simulink model "MSFartoystyring"  (R2019a)
settings: Solver=ode45  StartTime=tstart  StopTime=tstop  RelTol=1e-3  EnableMultiTasking=on
values from neighbouring files (symbols this model uses):
  c = 0    [run.m]
  p0 = zeros(2,1)    [run.m]
  psi0 = 0    [run.m]
  r0 = 0    [run.m]
  tsamp = 10    [run.m]
  v0 = [6.63 0]'    [run.m]
undefined symbols (not defined in the file or in its folder): dc_mode, delta_c, K_d_psi, K_d_u, K_i_psi, K_i_u, K_p_psi, K_p_u, k_reg, msfartoystyring, nc_mode, nc_step_final, nc_step_start, nc_step_time, psi_d_amp, psi_d_bias, psi_d_freq, r_reg, u_d_step_final, u_d_step_start, u_d_step_time
settings Model: ExtModeAutoUpdateStatusClock=off  Creator=christh  LastModifiedBy=paalthorseth
settings DataIOCC: LimitDataPoints=on  SaveFormat=Array  SignalLoggingSaveFormat=ModelDataLogs  ReturnWorkspaceOutputs=off
settings OptimizationCC: ExpressionDepthLimit=2147483647  InitFltsAndDblsToZero=on  LifeSpan=inf
settings DebuggingCC: UnderspecifiedInitializationDetection=Classic  MergeDetectMultiDrivingBlocksExec=none  SolverPrmCheckMsg=warning  FcnCallInpInsideContextMsg=warning  StateNameClashWarn=warning  SFUnexpectedBacktrackingDiag=warning  SFNoUnconditionalDefaultTransitionDiag=warning  ArithmeticOperatorsInVariantConditions=warning
settings HardwareCC: ProdBitPerPointer=32  ProdBitPerSizeT=32  ProdBitPerPtrDiffT=32  ProdLargestAtomicFloat=None  ProdIntDivRoundTo=Undefined  ProdEndianess=Unspecified  ProdWordSize=32  ProdHWDeviceType=32-bit Generic
settings ModelReferenceCC: PropagateSignalLabelsOutOfModel=off
settings SFSimCC: SimUseLocalCustomCode=off
settings RTWCC: RTWUseLocalCustomCode=off
settings CodeAppCC: StateflowObjectComments=on
settings GRTTargetCC: TargetLangStandard=C89/C90 (ANSI)  GeneratePreprocessorConditionals=Disable all  CombineOutputUpdateFcns=off  GRTInterface=on
settings ConfigComp: CovMetricSettings=dw  CovHtmlReporting=on  CovSaveCumulativeToWorkspaceVar=on  CovSaveSingleToWorkspaceVar=on  CovExternalEMLEnable=off

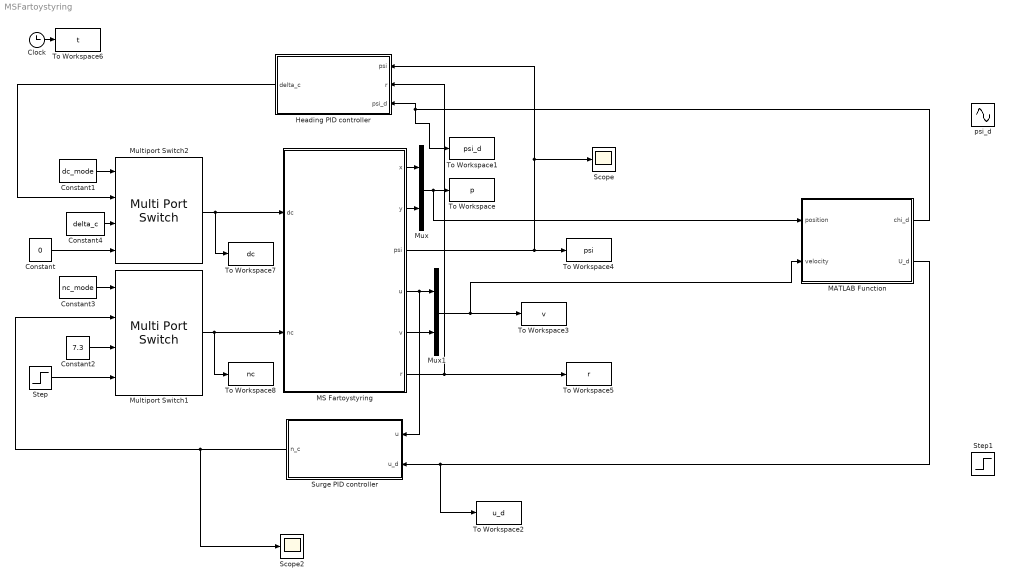
== system MSFartoystyring ==
  Clock : Clock
  Constant : Constant  Value=0
  Constant1 : Constant  Value=dc_mode
  Constant2 : Constant  Value=7.3
  Constant3 : Constant  Value=nc_mode
  Constant4 : Constant  Value=delta_c
  Heading PID controller : Subsystem
  MATLAB Function : MATLAB Function  TreatAsAtomicUnit=on  SystemSampleTime=0.1
  MS Fartoystyring : Subsystem  mask(MS Fartoystyring for Assignment 3 G&C){x0=p0(1), y0=p0(2), u0=v0(1), v0=v0(2), psi0=psi0, r0=r0, c=c}
      mask prompts: x0 "x(t0) (m)"; y0 "y(t0) (m)"; u0 "u(t0) (m/s)"; v0 "v(t0) (m/s)"; psi0 "psi(t0) (rad)"; r0 "r(t0) (rad/s)"; c "current (0 or 1)"
      mask help:
      | Block corresponding to Figure 1 in the assignment text. Gives the response of the ship.
      |
      | The design speed of MS Fartoystyring is u=8.23 m/s.
      |
      | Input:
      | dc: commanded rudder (rad), dmax=25*pi/180
      | nc: commanded shaft speed (rad/s), nmax=85*2*pi/60
      |
      | Output:
      | x: north pos (m)
      | y: east pos (m)
      | u: surge (m/s)
      | v: sway (m/s)
      | psi: heading (rad)
      | r: yaw (rad/s)
      mask Help: Comments, bugs and help requests can be directed to the TA. Email on course website.
  Multiport Switch1 : MultiPortSwitch  DataPortOrder=Specify indices  DataPortIndices={NC_MODE.CONTROLLER, NC_MODE.CONSTANT, NC_MODE.STEP}  DiagnosticForDefault=None
  Multiport Switch2 : MultiPortSwitch  DataPortOrder=Specify indices  DataPortIndices={DC_MODE.CONTROLLER, DC_MODE.CONSTANT, DC_MODE.ZERO}
  Mux : Mux  Inputs=2
  Mux1 : Mux  Inputs=2
  Scope : Scope
  Scope2 : Scope
  Step : Step  Time=nc_step_time  Before=nc_step_start  After=nc_step_final  SampleTime=0
  Step1 : Step  Time=u_d_step_time  Before=u_d_step_start  After=u_d_step_final  SampleTime=0
  Surge PID controller : Subsystem
  To Workspace : ToWorkspace  VariableName=p  SampleTime=tsamp
  To Workspace1 : ToWorkspace  VariableName=psi_d  SampleTime=tsamp
  To Workspace2 : ToWorkspace  VariableName=u_d  SampleTime=tsamp
  To Workspace3 : ToWorkspace  VariableName=v  SampleTime=tsamp
  To Workspace4 : ToWorkspace  VariableName=psi  SampleTime=tsamp
  To Workspace5 : ToWorkspace  VariableName=r  SampleTime=tsamp
  To Workspace6 : ToWorkspace  VariableName=t  SampleTime=tsamp
  To Workspace7 : ToWorkspace  VariableName=dc  SampleTime=tsamp
  To Workspace8 : ToWorkspace  VariableName=nc  SampleTime=tsamp
  psi_d : Sin  Amplitude=psi_d_amp  Bias=psi_d_bias  Frequency=psi_d_freq  SampleTime=0
  wires:
  Clock/1 -> To Workspace6/1
  MS Fartoystyring/1(x) -> Mux/1
  MS Fartoystyring/2(y) -> Mux/2
  MS Fartoystyring/5(v) -> Mux1/2
  MS Fartoystyring/3(psi) -> To Workspace4/1, Heading PID controller/1(psi), Scope/1
  MS Fartoystyring/6(r) -> To Workspace5/1, Heading PID controller/2(r)
  MATLAB Function/1(chi_d) -> To Workspace1/1, Heading PID controller/3(psi_d)
  Step/1 -> Multiport Switch1/4
  Constant2/1 -> Multiport Switch1/3
  Constant1/1 -> Multiport Switch2/1
  Constant3/1 -> Multiport Switch1/1
  Constant/1 -> Multiport Switch2/4
  Constant4/1 -> Multiport Switch2/3
  Heading PID controller/1(delta_c) -> Multiport Switch2/2
  Surge PID controller/1(n_c) -> Scope2/1, Multiport Switch1/2
  Multiport Switch2/1 -> To Workspace7/1, MS Fartoystyring/1(dc)
  Multiport Switch1/1 -> MS Fartoystyring/2(nc), To Workspace8/1
  MATLAB Function/2(U_d) -> Surge PID controller/2(u_d), To Workspace2/1
  MS Fartoystyring/4(u) -> Surge PID controller/1(u), Mux1/1
  Mux/1 -> MATLAB Function/1(position), To Workspace/1
  Mux1/1 -> MATLAB Function/2(velocity), To Workspace3/1

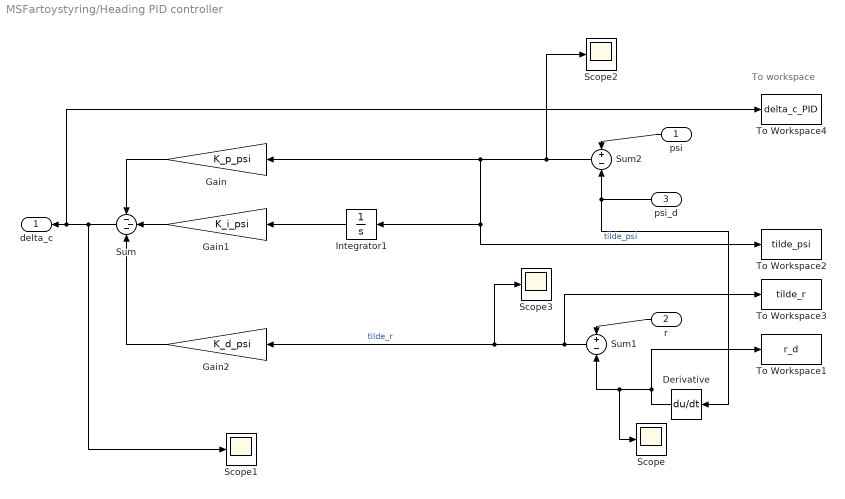
== system MSFartoystyring/Heading PID controller ==
  note: To workspace
  psi : Inport
  r : Inport  Port=2
  psi_d : Inport  Port=3
  Derivative : Derivative
  Gain : Gain  Gain=K_p_psi
  Gain1 : Gain  Gain=K_i_psi
  Gain2 : Gain  Gain=K_d_psi
  Integrator1 : Integrator
  Scope{,1..3} (4 alike) : Scope
  Sum : Sum  Inputs=---
  Sum1 : Sum  Inputs=+|-
  Sum2 : Sum  Inputs=+|-
  To Workspace1 : ToWorkspace  VariableName=r_d  SampleTime=tsamp
  To Workspace2 : ToWorkspace  VariableName=tilde_psi  SampleTime=tsamp
  To Workspace3 : ToWorkspace  VariableName=tilde_r  SampleTime=tsamp
  To Workspace4 : ToWorkspace  VariableName=delta_c_PID  SampleTime=tsamp
  delta_c : Outport
  wires:
  Sum/1 -> Scope1/1, delta_c/1, To Workspace4/1
  Gain/1 -> Sum/1
  Sum2/1 -> Scope2/1, Integrator1/1, To Workspace2/1, Gain/1  "tilde_psi"
  Derivative/1 -> Scope/1, Sum1/2, To Workspace1/1
  Integrator1/1 -> Gain1/1
  r/1 -> Sum1/1
  Sum1/1 -> Scope3/1, Gain2/1, To Workspace3/1  "tilde_r"
  psi/1 -> Sum2/1
  psi_d/1 -> Derivative/1, Sum2/2
  Gain2/1 -> Sum/3
  Gain1/1 -> Sum/2

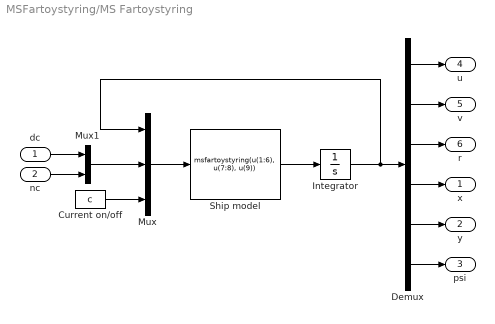
== system MSFartoystyring/MS Fartoystyring ==
  dc : Inport
  nc : Inport  Port=2
  Current on/off : Constant  Value=c
  Demux : Demux  Outputs=6
  Integrator : Integrator  InitialCondition=[u0 v0 r0 x0 y0 psi0]'
  Mux : Mux  Inputs=3
  Mux1 : Mux  Inputs=2
  Ship model : MATLABFcn  MATLABFcn=msfartoystyring(u(1:6), u(7:8), u(9))  OutputDimensions=6
  x : Outport
  y : Outport  Port=2
  psi : Outport  Port=3
  u : Outport  Port=4
  v : Outport  Port=5
  r : Outport  Port=6
  wires:
  Integrator/1 -> Mux/1, Demux/1
  Mux1/1 -> Mux/2
  dc/1 -> Mux1/1
  nc/1 -> Mux1/2
  Demux/1 -> u/1
  Demux/2 -> v/1
  Demux/3 -> r/1
  Demux/4 -> x/1
  Demux/5 -> y/1
  Demux/6 -> psi/1
  Current on/off/1 -> Mux/3
  Ship model/1 -> Integrator/1
  Mux/1 -> Ship model/1

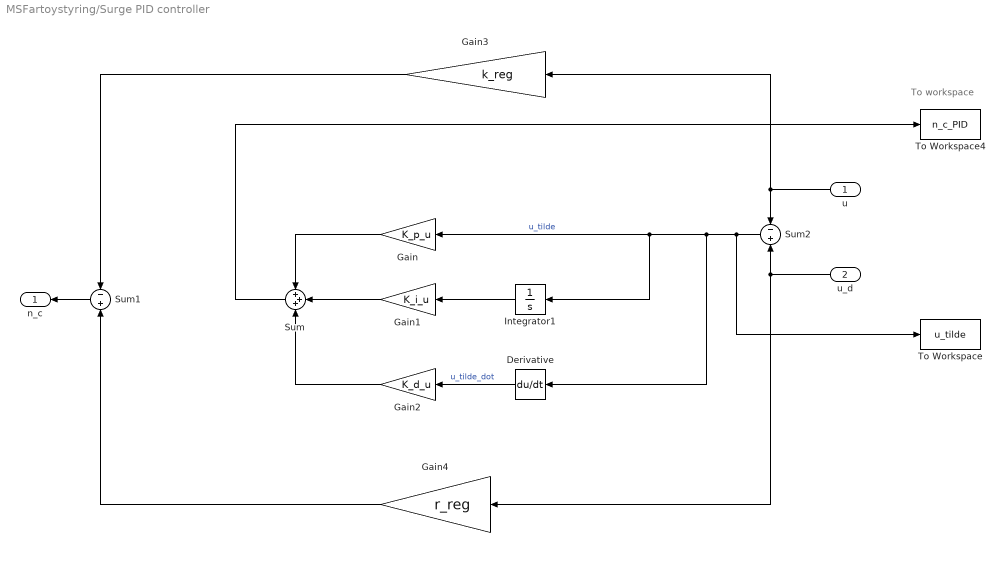
== system MSFartoystyring/Surge PID controller ==
  note: To workspace
  u : Inport
  u_d : Inport  Port=2
  Derivative : Derivative
  Gain : Gain  Gain=K_p_u
  Gain1 : Gain  Gain=K_i_u
  Gain2 : Gain  Gain=K_d_u
  Gain3 : Gain  Gain=k_reg
  Gain4 : Gain  Gain=r_reg
  Integrator1 : Integrator
  Sum : Sum  Inputs=+++
  Sum1 : Sum  Inputs=-+
  Sum2 : Sum  Inputs=-|+
  To Workspace : ToWorkspace  VariableName=u_tilde  SampleTime=tsamp
  To Workspace4 : ToWorkspace  VariableName=n_c_PID  SampleTime=tsamp
  n_c : Outport
  wires:
  Gain/1 -> Sum/1
  Sum2/1 -> Derivative/1, Integrator1/1, Gain/1, To Workspace/1  "u_tilde"
  Integrator1/1 -> Gain1/1
  Gain2/1 -> Sum/3
  Gain1/1 -> Sum/2
  Derivative/1 -> Gain2/1  "u_tilde_dot"
  u/1 -> Gain3/1, Sum2/1
  u_d/1 -> Gain4/1, Sum2/2
  Sum/1 -> To Workspace4/1
  Gain3/1 -> Sum1/1
  Gain4/1 -> Sum1/2
  Sum1/1 -> n_c/1

== matlab function MSFartoystyring/MATLAB Function ==
  data: position input; chi_d output; velocity input; U_d output
function [chi_d, U_d]= Lookahead_LOS_Guidance(position,velocity)

% Initializing
persistent init_flag n K_p S;

if isempty(init_flag)
    % Load waypoints
    S   = load('WP.mat');
    
    % Define waypoint number, n
    n   = 1;
    
    % Controller parameters
    Delta   = 10000;
    K_p     = 1/Delta;
    
    init_flag = 1;
end


% Define variables
x       = position(1);     % position x in NED
y       = position(2);     % position y in NED

u       = velocity(1);     % velocity u in BODY
v       = velocity(2);     % velocity v in BODY

% Current waypoint
x_wp_c  = S.WP(1,n);
y_wp_c  = S.WP(2,n);

% Next waypoint
x_wp_n  = S.WP(1,n+1);
y_wp_n  = S.WP(2,n+1);

% Path-tangential angle in [-pi,pi]
alpha   = atan2(y_wp_n - y_wp_c, x_wp_n - x_wp_c);

% Map alpha to [0,2pi)
if alpha < 0 
    alpha = 2*pi + alpha;
end

% Cross-track error
e       = - (x - x_wp_c)*sin(alpha) + (y - y_wp_c)*cos(alpha);

% Define course reference 
chi_p   = alpha;
chi_r   = atan(-K_p*e);
chi_d   = chi_p + chi_r;

% Radius for circle of acceptance
R       = 2*304.8; 

% Check circle of acceptance
if (((x_wp_n - x)^2 + (y_wp_n - y)^2) <= R^2) && (n < size(S.WP,2)-1)
    n       = n + 1;
end

% Set desired speed
U_d     = 3.5;            % [m/s]
